simulink model "Arduino_Deploy"  (R2019b)
settings: Solver=FixedStepAuto  StartTime=0.0  StopTime=10.0  RelTol=1e-3  EnableMultiTasking=on
libraries: arduinolib x1, arduinosensorlib x1
settings Model: SILPILModeSetting=veronly  ExtModeTrigDuration=2  Creator=Anas  LastModifiedBy=Anas
settings OptimizationCC: EnhancedBackFolding=on  PassReuseOutputArgsAs=Individual arguments  ZeroExternalMemoryAtStartup=off  ZeroInternalMemoryAtStartup=off  MaxStackSize=64  OptimizeBlockOrder=speed  DifferentSizesBufferReuse=on  OptimizationCustomize=off  EfficientTunableParamExpr=on
settings DebuggingCC: ParameterTunabilityLossMsg=error
settings HardwareCC: ProdBitPerInt=16  ProdBitPerPointer=16  ProdBitPerSizeT=16  ProdBitPerPtrDiffT=16  ProdLargestAtomicFloat=None  ProdWordSize=8  ProdHWDeviceType=Atmel->AVR
settings SFSimCC: MATLABDynamicMemAlloc=off
settings RTWCC: SystemTargetFile=ert.tlc  HardwareBoard=Arduino Uno  TLCOptions=-aInlineSetEventsForThisBaseRateFcn=TLC_FALSE -aSuppressMultiTaskScheduler=TLC_FALSE -aRateBasedStepFcn=1  TemplateMakefile=ert_default_tmf  GenerateReport=on  Toolchain=Arduino AVR  BuildConfiguration=Faster Runs  IncludeHyperlinkInReport=on  LaunchReport=on  GenerateTraceInfo=on  GenerateTraceReport=on  GenerateTraceReportSl=on  GenerateTraceReportSf=on  GenerateTraceReportEml=on
settings CodeAppCC: ForceParamTrailComments=on  IgnoreCustomStorageClasses=off  OperatorAnnotations=on  SimulinkDataObjDesc=on  SFDataObjDesc=on  InsertBlockDesc=on
settings ERTTargetCC: SupportContinuousTime=on  SupportVariableSizeSignals=on  ExtModeStaticAllocSize=250

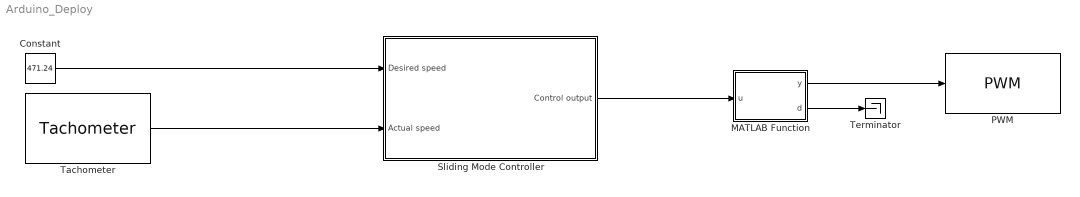
== system Arduino_Deploy ==
  Constant : Constant  Value=471.24
  MATLAB Function : MATLAB Function  TreatAsAtomicUnit=on
  PWM : arduinolib/PWM  pinNumber=5  EnableInputFrequency=off  InitialFrequency=2000  InitialDutyCycle=0  NotificationType=None  blockPlatform=arduino
  Sliding Mode Controller : Subsystem
  Tachometer : arduinosensorlib/Tachometer  PinNumber=2  InterruptMode=RISING  SampleTime=0.1  blockPlatform=ARDUINO
      settings: SourceProductName=Simulink Support Package for Arduino Hardware  SourceProductBaseCode=ARDUINO
  Terminator : Terminator
  wires:
  Tachometer/1 -> Sliding Mode Controller/2(Actual speed)
  Sliding Mode Controller/1(Control output) -> MATLAB Function/1(u)
  Constant/1 -> Sliding Mode Controller/1(Desired speed)
  MATLAB Function/1(y) -> PWM/1
  MATLAB Function/2(d) -> Terminator/1

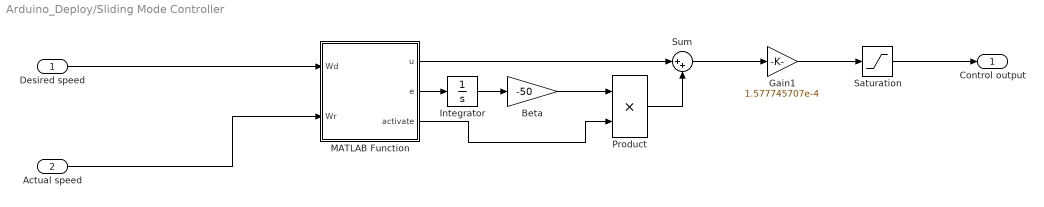
== system Arduino_Deploy/Sliding Mode Controller ==
  Desired speed : Inport
  Actual speed : Inport  Port=2
  Beta : Gain  Gain=-50
  Gain1 : Gain  Gain=1.577745707e-4
  Integrator : Integrator
  MATLAB Function : MATLAB Function  TreatAsAtomicUnit=on
  Product : Product
  Saturation : Saturate  UpperLimit=11  LowerLimit=-11
  Sum : Sum  Inputs=|++
  Control output : Outport
  wires:
  Actual speed/1 -> MATLAB Function/2(Wr)
  Gain1/1 -> Saturation/1
  Desired speed/1 -> MATLAB Function/1(Wd)
  Saturation/1 -> Control output/1
  MATLAB Function/2(e) -> Integrator/1
  Integrator/1 -> Beta/1
  Sum/1 -> Gain1/1
  MATLAB Function/1(u) -> Sum/1
  MATLAB Function/3(activate) -> Product/2
  Beta/1 -> Product/1
  Product/1 -> Sum/2

== matlab function Arduino_Deploy/MATLAB Function ==
  data: u input; y output; d output
function [y,d]= map(u)
if (u<0)
    d=0;
else
    d=1;
y = u/11*255;
end

== matlab function Arduino_Deploy/Sliding Mode Controller/MATLAB Function ==
  data: Wd input; u output; Wr input; e output; activate output
function [u,e,activate] = SMC(Wd,Wr)
%Sliding mode controller for a motor-propeller system
%Model
function y=f(x)
        y=-0.08653*x^2-39.902*x;
end
e=Wr-Wd;
mu=20;
Ku=6338.1;
static=Ku*8.6921948;
activate=1;
u=(-f(Wr)-Ku*mu*sign(e)*sqrt(abs(e)))*activate+static*(1-activate);
end
